simulink model "qhkz"  (Simulink 9.0)
settings: Solver=ode23tb  StartTime=0.0  StopTime=5  MaxStep=1e-5  RelTol=1e-4  EnableMultiTasking=on
undefined symbols (not defined in the file or in its folder): sigbuilder_block
libraries: powerlib x22, simulink x1
settings Model: Creator=Administrator  LastModifiedBy=dell
settings SolverCC: ZeroCrossAlgorithm=Adaptive  AlgebraicLoopSolver=LineSearch
settings DataIOCC: LimitDataPoints=on  SignalLoggingSaveFormat=ModelDataLogs
settings OptimizationCC: ExpressionDepthLimit=2147483647
settings DebuggingCC: MaxConsecutiveZCsMsg=none  SolverPrmCheckMsg=warning  FcnCallInpInsideContextMsg=warning  StateNameClashWarn=warning
settings GRTTargetCC: GeneratePreprocessorConditionals=Disable all  CombineOutputUpdateFcns=off  GRTInterface=on

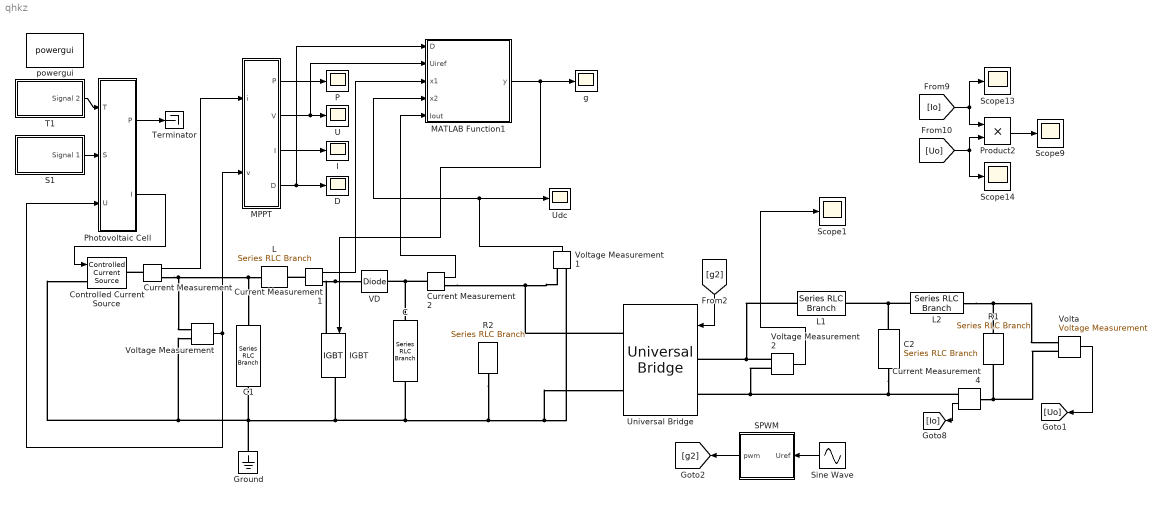
== system qhkz ==
  C : powerlib/Elements/Series RLC Branch  LConnTagsString=__new0  RConnTagsString=__new0  BranchType=C  Resistance=0  Inductance=0  SetiL0=off  InitialCurrent=0  Capacitance=300e-6  Setx0=on  InitialVoltage=0  Measurements=None
  C1 : powerlib/Elements/Series RLC Branch  LConnTagsString=__new0  RConnTagsString=__new0  BranchType=C  Resistance=0  Inductance=0  SetiL0=off  InitialCurrent=0  Capacitance=300e-5  Setx0=off  InitialVoltage=0  Measurements=None
  C2 : powerlib/Elements/Series RLC Branch  LConnTagsString=__new0  RConnTagsString=__new0  BranchType=C  Resistance=1  Inductance=1e-3  SetiL0=off  InitialCurrent=0  Capacitance=20e-6  Setx0=off  InitialVoltage=0  Measurements=None
  Controlled Current Source : powerlib/Electrical Sources/Controlled Current Source  Initialize=on  Source_Type=DC  Amplitude=0  Phase=0  Frequency=0  Measurements=None
  Current Measurement{,1..2,4} (4 alike) : powerlib/Measurements/Current Measurement  PhasorSimulation=off  OutputType=Complex  PSBequivalent=0
  D : Scope
  Ground : powerlib/Elements/Ground  LConnTagsString=a
  I : Scope
  IGBT : powerlib/Power Electronics/IGBT  Ron=0.00000001  Lon=0  Vf=0  Tf=1e-6  Tt=2e-6  IC=0  Rs=1e5  Cs=inf  Measurements=off
  L : powerlib/Elements/Series RLC Branch  LConnTagsString=__new0  RConnTagsString=__new0  BranchType=L  Resistance=0  Inductance=1e-3  SetiL0=off  InitialCurrent=1  Capacitance=inf  Setx0=off  InitialVoltage=0  Measurements=None
  L1 : powerlib/Elements/Series RLC Branch  LConnTagsString=__new0  RConnTagsString=__new0  BranchType=L  Resistance=1  Inductance=3e-3  SetiL0=off  InitialCurrent=0  Capacitance=1e-6  Setx0=off  InitialVoltage=0  Measurements=None
  L2 : powerlib/Elements/Series RLC Branch  LConnTagsString=__new0  RConnTagsString=__new0  BranchType=L  Resistance=1  Inductance=1e-3  SetiL0=off  InitialCurrent=0  Capacitance=1e-6  Setx0=off  InitialVoltage=0  Measurements=None
  MATLAB Function1 : MATLAB Function  TreatAsAtomicUnit=on
  MPPT : Subsystem
  P : Scope
  Photovoltaic Cell : Subsystem  mask(Photovoltaic Cell){a=0.00398, b=0.0821, Rs=0.5, Isc=1, Uoc=21.7, Im=0.91, Um=17.6, Sref=1000, Tref=25}
  Product2 : Product
  R1 : powerlib/Elements/Series RLC Branch  LConnTagsString=__new0  RConnTagsString=__new0  BranchType=R  Resistance=100  Inductance=1e-3  SetiL0=off  InitialCurrent=0  Capacitance=1e-6  Setx0=off  InitialVoltage=0  Measurements=None
  R2 : powerlib/Elements/Series RLC Branch  LConnTagsString=__new0  RConnTagsString=__new0  BranchType=R  Resistance=100  Inductance=1e-3  SetiL0=off  InitialCurrent=0  Capacitance=1e-6  Setx0=off  InitialVoltage=0  Measurements=None
  S1 : Subsystem  Tag=STV Subsys  LoadFcn=sigbuilder_block('load');  StartFcn=sigbuilder_block('start');  StopFcn=sigbuilder_block('stop');  ClipboardFcn=sigbuilder_block('clipboard');  mask(Sigbuilder block){tuvar=[0:10]}
      mask help: Sigbuilder GUI
      mask init:
      | if ~strcmp(get_param(bdroot(gcbh),'SimulationStatus'),'stopped') tuvar = sigbuilder_block('maskInit'); end
      settings: CopyFcn=sigbuilder_block('copy');  DeleteFcn=sigbuilder_block('delete');  ModelCloseFcn=sigbuilder_block('modelClose');  PreSaveFcn=sigbuilder_block('preSave');  PauseFcn=sigbuilder_block('pause')  ContinueFcn=sigbuilder_block('continue')  NameChangeFcn=sigbuilder_block('namechange');  OpenFcn=sigbuilder_block('open',[50.2759 41.5862 518.897 397.241 ]);  CloseFcn=sigbuilder_block('close');
      mask Display: plot(0, 0, 100, 100,[2, 2, 32, 32, 2], [68, 8, 8, 68, 68],[32, 2], [38, 38], [32, 19, 2],[53, 60, 44], [32, 17, 17, 2],[16, 16, 31, 31]);txt = getActiveGroup(gcbh);text(2, 100, txt,'verticalAlignment', 'top');
  SPWM : Subsystem
  Scope{1,9,13..14} (4 alike) : Scope
  Sine Wave : Sin  Frequency=100*pi  SampleTime=0
  T1 : Subsystem  Tag=STV Subsys  LoadFcn=sigbuilder_block('load');  StartFcn=sigbuilder_block('start');  StopFcn=sigbuilder_block('stop');  ClipboardFcn=sigbuilder_block('clipboard');  mask(Sigbuilder block){tuvar=[0:10]}
      mask help: Sigbuilder GUI
      mask init:
      | if ~strcmp(get_param(bdroot(gcbh),'SimulationStatus'),'stopped') tuvar = sigbuilder_block('maskInit'); end
      settings: CopyFcn=sigbuilder_block('copy');  DeleteFcn=sigbuilder_block('delete');  ModelCloseFcn=sigbuilder_block('modelClose');  PreSaveFcn=sigbuilder_block('preSave');  PauseFcn=sigbuilder_block('pause')  ContinueFcn=sigbuilder_block('continue')  NameChangeFcn=sigbuilder_block('namechange');  OpenFcn=sigbuilder_block('open',[142.759 39.1034 519.517 399.724 ]);  CloseFcn=sigbuilder_block('close');
      mask Display: plot(0, 0, 100, 100,[2, 2, 32, 32, 2], [68, 8, 8, 68, 68],[32, 2], [38, 38], [32, 19, 2],[53, 60, 44], [32, 17, 17, 2],[16, 16, 31, 31]);txt = getActiveGroup(gcbh);text(2, 100, txt,'verticalAlignment', 'top');
  Terminator : Terminator
  U : Scope
  Udc : Scope
  Universal Bridge : powerlib/Power Electronics/Universal Bridge  Arms=2  SnubberResistance=1e5  SnubberCapacitance=inf  Device=IGBT / Diodes  Ron=1e-6  Lon=0  ForwardVoltages="[  0  0  ]"  ForwardVoltage=0  GTOparameters=[ 10e-6 , 20e-6 ]  IGBTparameters=[ 1e-6 , 2e-6 ]  Measurements=None  Measurements_2=None  converterType=Rectifier
  VD : powerlib/Power Electronics/Diode  Ron=0.00000001  Lon=0  Vf=0  IC=0  UseSnubber=off  Rs=500  Cs=250e-9  Measurements=off
  Volta : powerlib/Measurements/Voltage Measurement  PhasorSimulation=off  OutputType=Complex  PSBequivalent=0
  Voltage Measurement : powerlib/Measurements/Voltage Measurement  PhasorSimulation=off  OutputType=Complex  PSBequivalent=0
  Voltage Measurement1 : powerlib/Measurements/Voltage Measurement  PhasorSimulation=off  OutputType=Complex  PSBequivalent=0
  Voltage Measurement2 : powerlib/Measurements/Voltage Measurement  PhasorSimulation=off  OutputType=Complex  PSBequivalent=0
  g : Scope
  powergui : powerlib/powergui  Priority=1  SimulationMode=Continuous  SampleTime=50e-8  frequency=60  Iterations=50  frequencyindice=0  Pbase=100e6  ErrMax=1e-4  UnitsV=kV  UnitsW=MW  buscounter=0  FunctionMessages=off  echomessages=off  EnableUseOfTLC=off  CurrentSourceSwitches=off  DisableSnubberDevices=off  DisableRonSwitches=off  DisableVfSwitches=off  DisplayEquations=off  SolverType=Tustin/Backward Euler (TBE)  Interpol=off  ExternalGateDelay=off  methode=off  Ts=100  x0status=blocks  SPID=off  SwTol=0  HookPort=off  RestoreLinks=warning  ResistiveCurrentMeasurement=off  Frange=[0:2:500]  Ylog=off  Xlog=on  ShowGrid=off  save=off  variable=ZData  structure=0  ZoomFFT=off  StartTime=0.0  cycles=1  DisplayStyle=1  fundamental=60  FreqAxis=off  MaxFrequency=1000  frequencyindicesteady=1  RmsSteady=1  display=off
  wires:
  Photovoltaic Cell/2(I) -> Controlled Current Source/1
  Voltage Measurement/1 -> Photovoltaic Cell/3(U), MPPT/2(v)
  Photovoltaic Cell/1(P) -> Terminator/1
  T1/1(Signal 2) -> Photovoltaic Cell/1(T)
  S1/1(Signal 1) -> Photovoltaic Cell/2(S)
  Current Measurement/1 -> MPPT/1(i)
  MPPT/1(P) -> P/1
  MPPT/3(I) -> I/1
  MPPT/2(V) -> MATLAB Function1/2(Uiref), U/1
  Voltage Measurement1/1 -> Udc/1, MATLAB Function1/4(x2)
  Current Measurement1/1 -> MATLAB Function1/3(x1)
  MPPT/4(D) -> MATLAB Function1/1(D), D/1
  MATLAB Function1/1(y) -> IGBT/1, g/1
  Current Measurement2/1 -> MATLAB Function1/5(Iout)
  [g2] -> Universal Bridge/1
  [Uo] -> Product2/2, Scope14/1
  Product2/1 -> Scope9/1
  Sine Wave/1 -> SPWM/1(Uref)
  Current Measurement4/1 -> [Io]
  SPWM/1(pwm) -> [g2]
  [Io] -> Product2/1, Scope13/1
  Volta/1 -> [Uo]
  Voltage Measurement2/1 -> Scope1/1
  connections:
  IGBT/LConn1 -- VD/LConn1 -- Current Measurement1/RConn1
  C/LConn1 -- Current Measurement2/LConn1 -- VD/RConn1
  Voltage Measurement/LConn1 -- Current Measurement/RConn1 -- C1/LConn1 -- L/LConn1
  C1/RConn1 -- Controlled Current Source/LConn1 -- Voltage Measurement/LConn2 -- Ground/LConn1 -- Universal Bridge/RConn2 -- Voltage Measurement1/LConn2 -- R2/RConn1 -- C/RConn1 -- IGBT/RConn1
  Current Measurement/LConn1 -- Controlled Current Source/RConn1
  Current Measurement1/LConn1 -- L/RConn1
  Current Measurement4/RConn1 -- C2/RConn1 -- Voltage Measurement2/LConn2 -- Universal Bridge/LConn2
  Current Measurement4/LConn1 -- Volta/LConn2 -- R1/RConn1
  Voltage Measurement2/LConn1 -- L1/LConn1 -- Universal Bridge/LConn1
  R1/LConn1 -- L2/RConn1 -- Volta/LConn1
  Current Measurement2/RConn1 -- Universal Bridge/RConn1 -- Voltage Measurement1/LConn1
  C2/LConn1 -- L2/LConn1 -- L1/RConn1

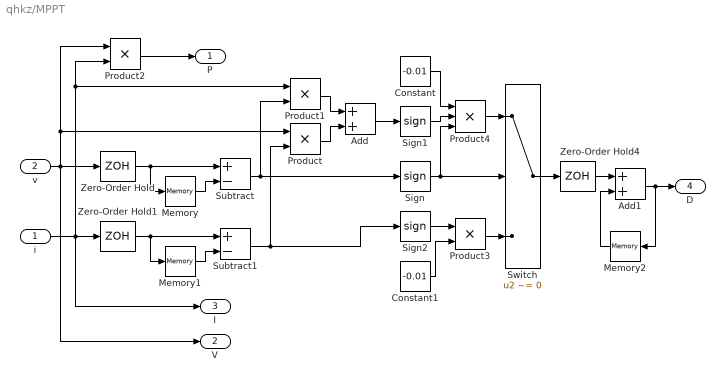
== system qhkz/MPPT ==
  i : Inport
  v : Inport  Port=2
  Add : Sum
  Add1 : Sum
  Constant : Constant  Value=-0.01
  Constant1 : Constant  Value=-0.01
  Memory : Memory
  Memory1 : Memory
  Memory2 : Memory  InitialCondition=1  InheritSampleTime=on
  Product{,1..3} (4 alike) : Product  RndMeth=Zero
  Product4 : Product  Inputs=3  RndMeth=Zero
  Sign : Signum
  Sign1 : Signum
  Sign2 : Signum
  Subtract : Sum  Inputs=+-
  Subtract1 : Sum  Inputs=+-
  Switch : Switch  Criteria=u2 ~= 0
  Zero-Order Hold : ZeroOrderHold  SampleTime=0.0005
  Zero-Order Hold1 : ZeroOrderHold  SampleTime=0.0005
  Zero-Order Hold4 : ZeroOrderHold  SampleTime=0.0005
  P : Outport
  V : Outport  Port=2
  I : Outport  Port=3
  D : Outport  Port=4
  wires:
  Memory2/1 -> Add1/2
  Add1/1 -> D/1, Memory2/1
  Product3/1 -> Switch/3
  Sign/1 -> Switch/2, Product4/3
  Constant1/1 -> Product3/2
  Sign2/1 -> Product3/1
  Constant/1 -> Product4/1
  Sign1/1 -> Product4/2
  Product1/1 -> Add/1
  Product/1 -> Add/2
  Subtract1/1 -> Product/2, Sign2/1
  Product2/1 -> P/1
  Subtract/1 -> Sign/1, Product1/2
  Memory1/1 -> Subtract1/2
  Zero-Order Hold1/1 -> Memory1/1, Subtract1/1
  i/1 -> Product2/2, Product1/1, I/1, Zero-Order Hold1/1
  Memory/1 -> Subtract/2
  Zero-Order Hold/1 -> Memory/1, Subtract/1
  v/1 -> Product/1, Product2/1, V/1, Zero-Order Hold/1
  Zero-Order Hold4/1 -> Add1/1
  Add/1 -> Sign1/1
  Product4/1 -> Switch/1
  Switch/1 -> Zero-Order Hold4/1

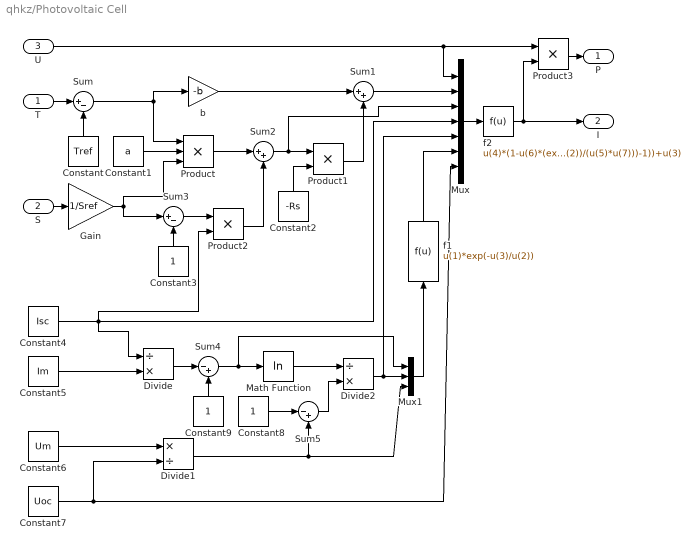
== system qhkz/Photovoltaic Cell ==
  T : Inport
  S : Inport  Port=2
  U : Inport  Port=3
  Constant : Constant  Value=Tref
  Constant1 : Constant  Value=a
  Constant2 : Constant  Value=-Rs
  Constant3 : Constant
  Constant4 : Constant  Value=Isc
  Constant5 : Constant  Value=Im
  Constant6 : Constant  Value=Um
  Constant7 : Constant  Value=Uoc
  Constant8 : Constant
  Constant9 : Constant
  Divide : Product  Inputs=/*
  Divide1 : Product  Inputs=*/
  Divide2 : Product  Inputs=/*
  Gain : Gain  Gain=1/Sref
  Math Function : Math  Operator=log  SaturateOnIntegerOverflow=on
  Mux : Mux  Inputs=7
  Mux1 : Mux  Inputs=3
  Product : Product  Inputs=3  RndMeth=Zero
  Product1 : Product  RndMeth=Zero
  Product2 : Product  RndMeth=Zero
  Product3 : Product  RndMeth=Zero
  Sum : Sum  Inputs=|+-
  Sum1 : Sum  Inputs=|++
  Sum2 : Sum  Inputs=|++
  Sum3 : Sum  Inputs=|+-
  Sum4 : Sum  Inputs=|-+
  Sum5 : Sum  Inputs=|-+
  b : Gain  Gain=-b
  f1 : Fcn  Expr=u(1)*exp(-u(3)/u(2))
  f2 : Fcn  Expr=u(4)*(1-u(6)*(exp((u(1)-u(2))/(u(5)*u(7)))-1))+u(3)
  P : Outport
  I : Outport  Port=2
  wires:
  T/1 -> Sum/1
  Sum/1 -> Product/1, b/1
  b/1 -> Sum1/1
  Constant/1 -> Sum/2
  S/1 -> Gain/1
  Gain/1 -> Product/3, Sum3/1
  Constant1/1 -> Product/2
  Product/1 -> Sum2/1
  Sum2/1 -> Product1/1, Mux/3
  Constant2/1 -> Product1/2
  Sum3/1 -> Product2/1
  Product2/1 -> Sum2/2
  Constant3/1 -> Sum3/2
  Product1/1 -> Sum1/2
  Constant4/1 -> Product2/2, Mux/4, Divide/1
  Sum1/1 -> Mux/2
  U/1 -> Mux/1, Product3/1
  Divide/1 -> Sum4/1
  Constant9/1 -> Sum4/2
  Constant5/1 -> Divide/2
  Constant7/1 -> Divide1/2, Mux/7
  Constant6/1 -> Divide1/1
  Sum4/1 -> Math Function/1, Mux1/1
  Divide1/1 -> Sum5/2, Mux1/3
  Constant8/1 -> Sum5/1
  Sum5/1 -> Divide2/2
  Math Function/1 -> Divide2/1
  Divide2/1 -> Mux1/2, Mux/5
  Mux1/1 -> f1/1
  f1/1 -> Mux/6
  Mux/1 -> f2/1
  Product3/1 -> P/1
  f2/1 -> I/1, Product3/2

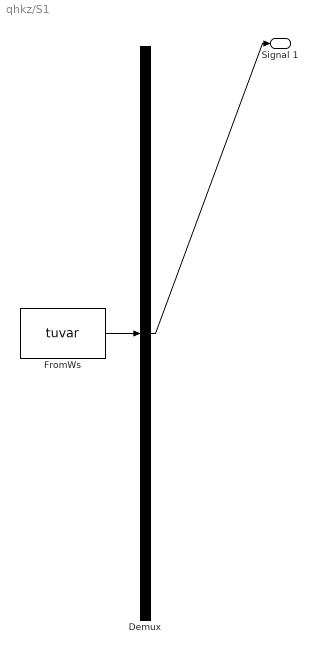
== system qhkz/S1 ==
  Demux : Demux  Tag=STV Demux  Outputs=1
  FromWs : FromWorkspace  Tag=STV FromWs  VariableName=tuvar  SampleTime=0  SigBuilderData=DataTag0  VnvData=DataTag1
      SigBuilderData=|
      | dataSet.timeRange = [0 0.16]
      | dataSet.name = 'Group 1'
      | sbobj.Groups.Name = 'Group 1'
      | sbobj.Groups.Signals.Name = 'Signal 1'
      | sbobj.Groups.Signals.XData = [0 0.05 0.16]
      | sbobj.Groups.Signals.YData = [1000 1000 1000]
      | sbobj.Groups.TimeRange = [0 0.16]
  Signal 1 : Outport  Tag=STV Outport
  wires:
  Demux/1 -> Signal 1/1
  FromWs/1 -> Demux/1

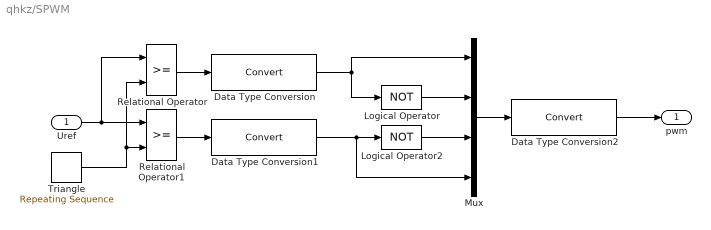
== system qhkz/SPWM ==
  Uref : Inport
  Data Type Conversion : DataTypeConversion
  Data Type Conversion1 : DataTypeConversion
  Data Type Conversion2 : DataTypeConversion
  Logical Operator : Logic  Operator=NOT  AllPortsSameDT=off  OutDataTypeStr=boolean
  Logical Operator2 : Logic  Operator=NOT  AllPortsSameDT=off  OutDataTypeStr=boolean
  Mux : Mux
  Relational Operator : RelationalOperator  RndMeth=Nearest  InputSameDT=on
  Relational Operator1 : RelationalOperator  RndMeth=Nearest  InputSameDT=on
  Triangle : simulink/Sources/Repeating Sequence  rep_seq_t=[0 1/5000/4 3/5000/4 1/5000]  rep_seq_y=[0 -1 1 0]
  pwm : Outport
  wires:
  Relational Operator1/1 -> Data Type Conversion1/1
  Relational Operator/1 -> Data Type Conversion/1
  Mux/1 -> Data Type Conversion2/1
  Uref/1 -> Relational Operator/1, Relational Operator1/1
  Triangle/1 -> Relational Operator/2, Relational Operator1/2
  Data Type Conversion/1 -> Logical Operator/1, Mux/1
  Logical Operator/1 -> Mux/2
  Data Type Conversion2/1 -> pwm/1
  Data Type Conversion1/1 -> Mux/4, Logical Operator2/1
  Logical Operator2/1 -> Mux/3

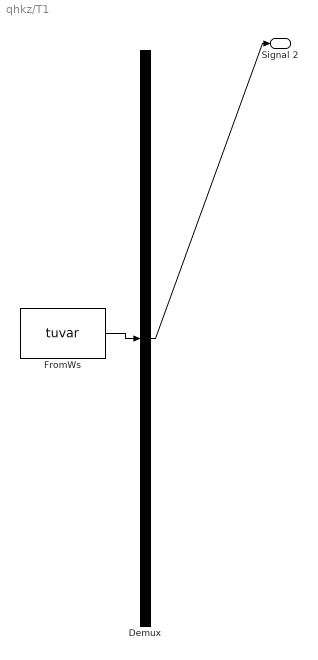
== system qhkz/T1 ==
  Demux : Demux  Tag=STV Demux  Outputs=1
  FromWs : FromWorkspace  Tag=STV FromWs  VariableName=tuvar  SampleTime=0  SigBuilderData=DataTag2  VnvData=DataTag3
      SigBuilderData=|
      | dataSet.timeRange = [0 0.16]
      | dataSet.name = 'Group 1'
      | sbobj.Groups.Name = 'Group 1'
      | sbobj.Groups.Signals.Name = 'Signal 2'
      | sbobj.Groups.Signals.XData = [0 0.1 0.16]
      | sbobj.Groups.Signals.YData = [25 25 25]
      | sbobj.Groups.TimeRange = [0 0.16]
  Signal 2 : Outport  Tag=STV Outport
  wires:
  FromWs/1 -> Demux/1
  Demux/1 -> Signal 2/1

== matlab function MATLAB Function1 ==
  data: D input double; Uiref input double; x1 input double; x2 input double; y output double; Iout input double
function y = fcn(D,Uiref,x1,x2,Iout)
%输出电压参考值
Uoref=Uiref/(1-D);
%负载值
R=x2/Iout;
%电感电流平均值
Id=Uoref^2/(R*Uiref);
%坐标平移
x01=x1-Id;
x02=x2-Uoref;
%Lyapnouv函数导数计算
%开关导通时（S=1)
v1=x01*(Uiref)+x02*Iout;
%开关关断时（S=0)
v2=x01*(Uiref-x2)+x02*(x1-Iout);
%开关切换规则
if v1<v2
    y=1;
else
    y=0;
end
